simulink model "lab4_41"  (R2023b)
settings: Solver=FixedStepAuto  StartTime=0.0  StopTime=10.0  FixedStep=0.001  RelTol=1e-3
undefined symbols (not defined in the file): A, k
settings Model: Creator=nsukh  LastModifiedBy=nsukh

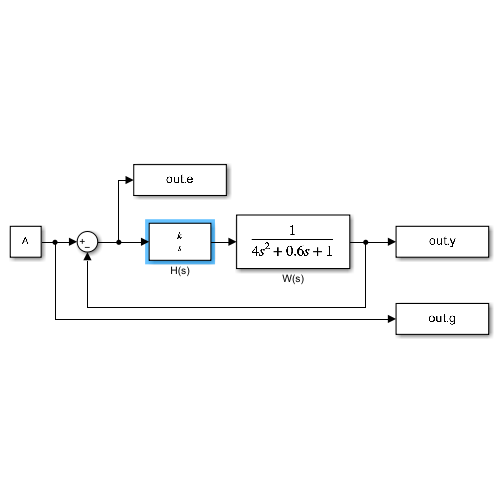
[thumbnail: Simulink's stored preview of the top-level diagram]
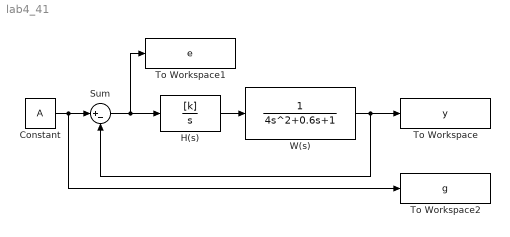
== system lab4_41 ==
  Constant : Constant  Value=A  SampleTime=-1
  H(s) : TransferFcn  Numerator=[k]  Denominator=[1 0]
  Sum : Sum  Inputs=|+-
  To Workspace : ToWorkspace  VariableName=y  SaveFormat=Timeseries  SampleTime=-1
  To Workspace1 : ToWorkspace  VariableName=e  SaveFormat=Timeseries  SampleTime=-1
  To Workspace2 : ToWorkspace  VariableName=g  SaveFormat=Timeseries  SampleTime=-1
  W(s) : TransferFcn  Denominator=[4 0.6 1]
  wires:
  H(s)/1 -> W(s)/1
  Sum/1 -> To Workspace1/1, H(s)/1
  W(s)/1 -> Sum/2, To Workspace/1
  Constant/1 -> To Workspace2/1, Sum/1
